simulink model "FFT_Analysis_Synthesis_VHDL"  (R2020a)
settings: Solver=FixedStepDiscrete  StartTime=0.0  StopTime=1  RelTol=1e-3
InitFcn:
  | sm_callback_init
StopFcn:
  | sm_callback_stop
values from neighbouring files (symbols this model uses):
  mp = sm_init_control_signals(mp)    [sm_callback_init.m]    (also in sm_callback_stop.m = sm_stop_verify(mp))
libraries: hdlsllib x32, simulink x12, dsphdlxfrm x4, dspsigops x2
(part 2 of 2)

== system FFT_Analysis_Synthesis_VHDL/dataplane/FFT_Analysis_Synthesis_Left/Analysis/FFT Frame Buffering/FFT_pulse_gen/Wait_for_data_to_start ==
  note: Frame pulses don't start
      | coming through until
      | circular buffer has data.
  note: Counter starts a zero and counts number of frame pulses.
      | Counter remains enabled while frame count is less than 4.
      | As soon as the counter reaches 4, it is disabled, which then
      | enables the frame pulses to pass through.
  note: Frame_Pulse
      | will pass through
      | when enabled
  note: Number of Frames
      | to wait before starting
  note: Start performing FFTs after enough data has filled the circular buffer.
      | This is due to the fact that we don't want the read pointer (addr_B)
      | to catch up with the write pointer (addr_A) because if it does,
      | the DPRAM will throw an assertion error.
  note: Enable signal that that indicates
      | that FFTs can start since there is
      | data in the buffer.
  Frame_Pulse : Inport
  Bitwise Operator : simulink/Logic and Bit Operations/Bitwise Operator  logicop=NOT  UseBitMask=off  BitMask=bin2dec('11011001')  BitMaskRealWorld=Stored Integer
  Compare To Constant : simulink/Logic and Bit Operations/Compare To Constant  relop=<  const=4  OutDataTypeStr=boolean
  Initial_frame_count : hdlsllib/Sources/HDL Counter  CountType=Count limited  CountInit=0  CountStep=1  CountMax=4  CountFromType=Specify  CountFrom=0  CountResetPort=off  CountLoadPort=off  CountEnbPort=on  CountDirPort=off  CountDataType=Unsigned  CountWordLen=5  CountFracLen=0  CountSampTime=1
  Logical Operator : Logic  AllPortsSameDT=off  OutDataTypeStr=boolean
  Logical Operator1 : Logic  AllPortsSameDT=off  OutDataTypeStr=boolean
  FFT_Frame_Start : Outport  VectorParamsAs1DForOutWhenUnconnected=off
  Enable_FFT_Frames : Outport  Port=2  VectorParamsAs1DForOutWhenUnconnected=off
  wires:
  Logical Operator1/1 -> FFT_Frame_Start/1
  Frame_Pulse/1 -> Logical Operator/2, Logical Operator1/1
  Initial_frame_count/1 -> Compare To Constant/1
  Logical Operator/1 -> Initial_frame_count/1
  Compare To Constant/1 -> Bitwise Operator/1, Logical Operator/1
  Bitwise Operator/1 -> Enable_FFT_Frames/1, Logical Operator1/2

== system FFT_Analysis_Synthesis_VHDL/dataplane/FFT_Analysis_Synthesis_Left/Analysis/FFT Frame Buffering/addr_B_gen/addr_B_gen_enable ==
  note: Signal that is enabled while
      | counting [0 FFT_size-1]
  note: Frame_index is the count [0 FFT_size-1]
      | that is used to lookup the window value
      | being applied to the streaming sample.
  note: This counter specifies where the FFT starts
      | in the circular buffer.  It increments by FFT/4
      | samples when it receives a start pulse.
  note: The start pulse resets the counter that counts
      | from zero to FFT_size-1.  Upon reaching FFT_size
      | the counter is disabled.  While the counter is enabled,
      | the enable signal tells the FFT engine that the data streaming
      | to it is valid.
  start : Inport
  B_Enable_Counter : hdlsllib/Sources/HDL Counter  CountType=Count limited  CountInit=0  CountStep=1  CountMax=mp.FFT_size  CountFromType=Specify  CountFrom=0  CountResetPort=on  CountLoadPort=off  CountEnbPort=on  CountDirPort=off  CountDataType=Unsigned  CountWordLen=mp.DPRAM1_address_size  CountFracLen=0  CountSampTime=1
  Constant5 : Constant  Value=mp.FFT_size  OutDataTypeStr=fixdt(0,mp.FFT_size_Nbits,0)  SampleTime=mp.Ts/mp.SysRate_Upsample_Factor
  Relational Operator : RelationalOperator  Operator=<=  OutDataTypeStr=boolean  ZeroCross=off  RndMeth=Nearest
  Start_Address_Counter : hdlsllib/Sources/HDL Counter  CountType=Free running  CountInit=0  CountStep=mp.FFT_frame_shift  CountMax=25  CountFromType=Initial value  CountFrom=0  CountResetPort=off  CountLoadPort=off  CountEnbPort=on  CountDirPort=off  CountDataType=Unsigned  CountWordLen=mp.DPRAM1_address_size  CountFracLen=0  CountSampTime=1
  enable_B : Outport  VectorParamsAs1DForOutWhenUnconnected=off
  Start_Address : Outport  Port=2  VectorParamsAs1DForOutWhenUnconnected=off
  Frame_Index : Outport  Port=3  VectorParamsAs1DForOutWhenUnconnected=off
  wires:
  Relational Operator/1 -> enable_B/1, B_Enable_Counter/2
  Constant5/1 -> Relational Operator/2
  B_Enable_Counter/1 -> Frame_Index/1, Relational Operator/1
  start/1 -> B_Enable_Counter/1, Start_Address_Counter/1
  Start_Address_Counter/1 -> Start_Address/1

== system FFT_Analysis_Synthesis_VHDL/dataplane/FFT_Analysis_Synthesis_Left/Frequency_Domain_Processing/Apply_Complex_Gains/FFT_Filter_Coefficients/FFT_ROM_Indexing ==
  note: When the index is FFT_size/2, we want the
      | index to be zero.
  note: Count from 0 to FFT_size
  note: Reverse direction of
      | count when count
      | is FFT_size/2
  note: Count from 0 to FFT_size/2 and then back down to 0.
      | We are assuming the gains are conjugate symmetric
      | so we only need to store the first half in the ROM
      | and look up again for negative frequencies.
  valid : Inport
  Bitwise Operator : simulink/Logic and Bit Operations/Bitwise Operator  logicop=NOT  UseBitMask=off  BitMask=bin2dec('11011001')  BitMaskRealWorld=Stored Integer
  Constant : Constant  Value=0  OutDataTypeStr=fixdt(0,mp.FFT_size_Nbits,0)  SampleTime=mp.Ts/mp.SysRate_Upsample_Factor
  Constant5 : Constant  Value=mp.FFT_size_half  OutDataTypeStr=fixdt(0,mp.FFT_size_Nbits,0)  SampleTime=mp.Ts/mp.SysRate_Upsample_Factor
  FFT_count : hdlsllib/Sources/HDL Counter  CountType=Free running  CountInit=0  CountStep=1  CountMax=25  CountFromType=Initial value  CountFrom=0  CountResetPort=on  CountLoadPort=off  CountEnbPort=on  CountDirPort=off  CountDataType=Unsigned  CountWordLen=mp.FFT_size_Nbits  CountFracLen=0  CountSampTime=1
  Relational Operator : RelationalOperator  Operator=<  OutDataTypeStr=boolean  ZeroCross=off  RndMeth=Nearest
  Relational Operator1 : RelationalOperator  Operator=~=  OutDataTypeStr=boolean  ZeroCross=off  RndMeth=Nearest
  Switch : Switch  Criteria=u2 > Threshold
  counter_gain_index : hdlsllib/Sources/HDL Counter  CountType=Free running  CountInit=0  CountStep=1  CountMax=25  CountFromType=Initial value  CountFrom=0  CountResetPort=on  CountLoadPort=off  CountEnbPort=on  CountDirPort=on  CountDataType=Unsigned  CountWordLen=mp.FFT_size_Nbits  CountFracLen=0  CountSampTime=1
  ROM_index : Outport
  wires:
  Relational Operator/1 -> counter_gain_index/3
  Bitwise Operator/1 -> FFT_count/1, counter_gain_index/1
  Relational Operator1/1 -> Switch/2
  FFT_count/1 -> Relational Operator/1
  valid/1 -> FFT_count/2, counter_gain_index/2, Bitwise Operator/1
  Constant5/1 -> Relational Operator1/2, Relational Operator/2
  counter_gain_index/1 -> Switch/1, Relational Operator1/1
  Constant/1 -> Switch/3
  Switch/1 -> ROM_index/1

== system FFT_Analysis_Synthesis_VHDL/dataplane/FFT_Analysis_Synthesis_Left/Frequency_Domain_Processing/Apply_Complex_Gains/FFT_Filter_Coefficients/Filter_ROM_Choice ==
  select : Inport
  Index : Inport  Port=2
  Complex_Gains_1_ROM : Subsystem
  Complex_Gains_2_ROM : Subsystem
  Complex_Gains_3_ROM : Subsystem
  Complex_Gains_4_ROM : Subsystem
  Multiport Switch : MultiPortSwitch  DataPortOrder=Zero-based contiguous  Inputs=4  zeroidx=on
  filter_gains : Outport
  wires:
  Multiport Switch/1 -> filter_gains/1
  Index/1 -> Complex_Gains_1_ROM/1(Index), Complex_Gains_2_ROM/1(Index), Complex_Gains_3_ROM/1(Index), Complex_Gains_4_ROM/1(Index)
  Complex_Gains_4_ROM/1(gains) -> Multiport Switch/5
  Complex_Gains_1_ROM/1(gains) -> Multiport Switch/2
  Complex_Gains_2_ROM/1(gains) -> Multiport Switch/3
  select/1 -> Multiport Switch/1
  Complex_Gains_3_ROM/1(gains) -> Multiport Switch/4

== system FFT_Analysis_Synthesis_VHDL/dataplane/FFT_Analysis_Synthesis_Right/Analysis/FFT Frame Buffering/FFT_pulse_gen/FFT_Frame_Pulse_Gen ==
  note: Create a FFT frame pulse that happens every FFT_size/4 samples.
      | We do this by watching when an appropriate subset of the counter bits
      | become zero.
  "counter_value " : Inport
  Bit Slice : hdlsllib/Logic and Bit Operations/Bit Slice  lidx=log2(mp.FFT_frame_shift)-1  ridx=0
      settings: SourceProductBaseCode=SL
  Compare To Zero : simulink/Logic and Bit Operations/Compare To Zero  relop===  OutDataTypeStr=boolean
  Frame_Pulse : Outport  VectorParamsAs1DForOutWhenUnconnected=off
  wires:
  "counter_value "/1 -> Bit Slice/1
  Compare To Zero/1 -> Frame_Pulse/1
  Bit Slice/1 -> Compare To Zero/1

== system FFT_Analysis_Synthesis_VHDL/dataplane/FFT_Analysis_Synthesis_Right/Analysis/FFT Frame Buffering/FFT_pulse_gen/Wait_for_data_to_start ==
  note: Frame pulses don't start
      | coming through until
      | circular buffer has data.
  note: Counter starts a zero and counts number of frame pulses.
      | Counter remains enabled while frame count is less than 4.
      | As soon as the counter reaches 4, it is disabled, which then
      | enables the frame pulses to pass through.
  note: Frame_Pulse
      | will pass through
      | when enabled
  note: Number of Frames
      | to wait before starting
  note: Start performing FFTs after enough data has filled the circular buffer.
      | This is due to the fact that we don't want the read pointer (addr_B)
      | to catch up with the write pointer (addr_A) because if it does,
      | the DPRAM will throw an assertion error.
  note: Enable signal that that indicates
      | that FFTs can start since there is
      | data in the buffer.
  Frame_Pulse : Inport
  Bitwise Operator : simulink/Logic and Bit Operations/Bitwise Operator  logicop=NOT  UseBitMask=off  BitMask=bin2dec('11011001')  BitMaskRealWorld=Stored Integer
  Compare To Constant : simulink/Logic and Bit Operations/Compare To Constant  relop=<  const=4  OutDataTypeStr=boolean
  Initial_frame_count : hdlsllib/Sources/HDL Counter  CountType=Count limited  CountInit=0  CountStep=1  CountMax=4  CountFromType=Specify  CountFrom=0  CountResetPort=off  CountLoadPort=off  CountEnbPort=on  CountDirPort=off  CountDataType=Unsigned  CountWordLen=5  CountFracLen=0  CountSampTime=1
  Logical Operator : Logic  AllPortsSameDT=off  OutDataTypeStr=boolean
  Logical Operator1 : Logic  AllPortsSameDT=off  OutDataTypeStr=boolean
  FFT_Frame_Start : Outport  VectorParamsAs1DForOutWhenUnconnected=off
  Enable_FFT_Frames : Outport  Port=2  VectorParamsAs1DForOutWhenUnconnected=off
  wires:
  Logical Operator1/1 -> FFT_Frame_Start/1
  Frame_Pulse/1 -> Logical Operator/2, Logical Operator1/1
  Initial_frame_count/1 -> Compare To Constant/1
  Logical Operator/1 -> Initial_frame_count/1
  Compare To Constant/1 -> Bitwise Operator/1, Logical Operator/1
  Bitwise Operator/1 -> Enable_FFT_Frames/1, Logical Operator1/2

== system FFT_Analysis_Synthesis_VHDL/dataplane/FFT_Analysis_Synthesis_Right/Analysis/FFT Frame Buffering/addr_B_gen/addr_B_gen_enable ==
  note: Signal that is enabled while
      | counting [0 FFT_size-1]
  note: Frame_index is the count [0 FFT_size-1]
      | that is used to lookup the window value
      | being applied to the streaming sample.
  note: This counter specifies where the FFT starts
      | in the circular buffer.  It increments by FFT/4
      | samples when it receives a start pulse.
  note: The start pulse resets the counter that counts
      | from zero to FFT_size-1.  Upon reaching FFT_size
      | the counter is disabled.  While the counter is enabled,
      | the enable signal tells the FFT engine that the data streaming
      | to it is valid.
  start : Inport
  B_Enable_Counter : hdlsllib/Sources/HDL Counter  CountType=Count limited  CountInit=0  CountStep=1  CountMax=mp.FFT_size  CountFromType=Specify  CountFrom=0  CountResetPort=on  CountLoadPort=off  CountEnbPort=on  CountDirPort=off  CountDataType=Unsigned  CountWordLen=mp.DPRAM1_address_size  CountFracLen=0  CountSampTime=1
  Constant5 : Constant  Value=mp.FFT_size  OutDataTypeStr=fixdt(0,mp.FFT_size_Nbits,0)  SampleTime=mp.Ts/mp.SysRate_Upsample_Factor
  Relational Operator : RelationalOperator  Operator=<=  OutDataTypeStr=boolean  ZeroCross=off  RndMeth=Nearest
  Start_Address_Counter : hdlsllib/Sources/HDL Counter  CountType=Free running  CountInit=0  CountStep=mp.FFT_frame_shift  CountMax=25  CountFromType=Initial value  CountFrom=0  CountResetPort=off  CountLoadPort=off  CountEnbPort=on  CountDirPort=off  CountDataType=Unsigned  CountWordLen=mp.DPRAM1_address_size  CountFracLen=0  CountSampTime=1
  enable_B : Outport  VectorParamsAs1DForOutWhenUnconnected=off
  Start_Address : Outport  Port=2  VectorParamsAs1DForOutWhenUnconnected=off
  Frame_Index : Outport  Port=3  VectorParamsAs1DForOutWhenUnconnected=off
  wires:
  Relational Operator/1 -> enable_B/1, B_Enable_Counter/2
  Constant5/1 -> Relational Operator/2
  B_Enable_Counter/1 -> Frame_Index/1, Relational Operator/1
  start/1 -> B_Enable_Counter/1, Start_Address_Counter/1
  Start_Address_Counter/1 -> Start_Address/1

== system FFT_Analysis_Synthesis_VHDL/dataplane/FFT_Analysis_Synthesis_Right/Frequency_Domain_Processing/Apply_Complex_Gains/FFT_Filter_Coefficients/FFT_ROM_Indexing ==
  note: When the index is FFT_size/2, we want the
      | index to be zero.
  note: Count from 0 to FFT_size
  note: Reverse direction of
      | count when count
      | is FFT_size/2
  note: Count from 0 to FFT_size/2 and then back down to 0.
      | We are assuming the gains are conjugate symmetric
      | so we only need to store the first half in the ROM
      | and look up again for negative frequencies.
  valid : Inport
  Bitwise Operator : simulink/Logic and Bit Operations/Bitwise Operator  logicop=NOT  UseBitMask=off  BitMask=bin2dec('11011001')  BitMaskRealWorld=Stored Integer
  Constant : Constant  Value=0  OutDataTypeStr=fixdt(0,mp.FFT_size_Nbits,0)  SampleTime=mp.Ts/mp.SysRate_Upsample_Factor
  Constant5 : Constant  Value=mp.FFT_size_half  OutDataTypeStr=fixdt(0,mp.FFT_size_Nbits,0)  SampleTime=mp.Ts/mp.SysRate_Upsample_Factor
  FFT_count : hdlsllib/Sources/HDL Counter  CountType=Free running  CountInit=0  CountStep=1  CountMax=25  CountFromType=Initial value  CountFrom=0  CountResetPort=on  CountLoadPort=off  CountEnbPort=on  CountDirPort=off  CountDataType=Unsigned  CountWordLen=mp.FFT_size_Nbits  CountFracLen=0  CountSampTime=1
  Relational Operator : RelationalOperator  Operator=<  OutDataTypeStr=boolean  ZeroCross=off  RndMeth=Nearest
  Relational Operator1 : RelationalOperator  Operator=~=  OutDataTypeStr=boolean  ZeroCross=off  RndMeth=Nearest
  Switch : Switch  Criteria=u2 > Threshold
  counter_gain_index : hdlsllib/Sources/HDL Counter  CountType=Free running  CountInit=0  CountStep=1  CountMax=25  CountFromType=Initial value  CountFrom=0  CountResetPort=on  CountLoadPort=off  CountEnbPort=on  CountDirPort=on  CountDataType=Unsigned  CountWordLen=mp.FFT_size_Nbits  CountFracLen=0  CountSampTime=1
  ROM_index : Outport
  wires:
  Relational Operator/1 -> counter_gain_index/3
  Bitwise Operator/1 -> FFT_count/1, counter_gain_index/1
  Relational Operator1/1 -> Switch/2
  FFT_count/1 -> Relational Operator/1
  valid/1 -> FFT_count/2, counter_gain_index/2, Bitwise Operator/1
  Constant5/1 -> Relational Operator1/2, Relational Operator/2
  counter_gain_index/1 -> Switch/1, Relational Operator1/1
  Constant/1 -> Switch/3
  Switch/1 -> ROM_index/1

== system FFT_Analysis_Synthesis_VHDL/dataplane/FFT_Analysis_Synthesis_Right/Frequency_Domain_Processing/Apply_Complex_Gains/FFT_Filter_Coefficients/Filter_ROM_Choice ==
  select : Inport
  Index : Inport  Port=2
  Complex_Gains_1_ROM : Subsystem
  Complex_Gains_2_ROM : Subsystem
  Complex_Gains_3_ROM : Subsystem
  Complex_Gains_4_ROM : Subsystem
  Multiport Switch : MultiPortSwitch  DataPortOrder=Zero-based contiguous  Inputs=4  zeroidx=on
  filter_gains : Outport
  wires:
  Multiport Switch/1 -> filter_gains/1
  Index/1 -> Complex_Gains_1_ROM/1(Index), Complex_Gains_2_ROM/1(Index), Complex_Gains_3_ROM/1(Index), Complex_Gains_4_ROM/1(Index)
  Complex_Gains_4_ROM/1(gains) -> Multiport Switch/5
  Complex_Gains_1_ROM/1(gains) -> Multiport Switch/2
  Complex_Gains_2_ROM/1(gains) -> Multiport Switch/3
  select/1 -> Multiport Switch/1
  Complex_Gains_3_ROM/1(gains) -> Multiport Switch/4

== system FFT_Analysis_Synthesis_VHDL/dataplane/FFT_Analysis_Synthesis_Left/Frequency_Domain_Processing/Apply_Complex_Gains/FFT_Filter_Coefficients/Filter_ROM_Choice/Complex_Gains_1_ROM ==
  Index : Inport
  Gains_ROM_imag : Subsystem
  Gains_ROM_real : Subsystem
  Real-Imag to Complex : RealImagToComplex
  gains : Outport
  wires:
  Gains_ROM_imag/1(gain_value_imag) -> Real-Imag to Complex/2
  Index/1 -> Gains_ROM_imag/1(Index), Gains_ROM_real/1(Index)
  Gains_ROM_real/1(gain_value_real) -> Real-Imag to Complex/1
  Real-Imag to Complex/1 -> gains/1

== system FFT_Analysis_Synthesis_VHDL/dataplane/FFT_Analysis_Synthesis_Left/Frequency_Domain_Processing/Apply_Complex_Gains/FFT_Filter_Coefficients/Filter_ROM_Choice/Complex_Gains_2_ROM ==
  Index : Inport
  Gains_ROM_imag : Subsystem
  Gains_ROM_real : Subsystem
  Real-Imag to Complex : RealImagToComplex
  gains : Outport
  wires:
  Gains_ROM_imag/1(gain_value_imag) -> Real-Imag to Complex/2
  Index/1 -> Gains_ROM_imag/1(Index), Gains_ROM_real/1(Index)
  Gains_ROM_real/1(gain_value_real) -> Real-Imag to Complex/1
  Real-Imag to Complex/1 -> gains/1

== system FFT_Analysis_Synthesis_VHDL/dataplane/FFT_Analysis_Synthesis_Left/Frequency_Domain_Processing/Apply_Complex_Gains/FFT_Filter_Coefficients/Filter_ROM_Choice/Complex_Gains_3_ROM ==
  Index : Inport
  Gains_ROM_imag : Subsystem
  Gains_ROM_real : Subsystem
  Real-Imag to Complex : RealImagToComplex
  gains : Outport
  wires:
  Gains_ROM_imag/1(gain_value_imag) -> Real-Imag to Complex/2
  Index/1 -> Gains_ROM_imag/1(Index), Gains_ROM_real/1(Index)
  Gains_ROM_real/1(gain_value_real) -> Real-Imag to Complex/1
  Real-Imag to Complex/1 -> gains/1

== system FFT_Analysis_Synthesis_VHDL/dataplane/FFT_Analysis_Synthesis_Left/Frequency_Domain_Processing/Apply_Complex_Gains/FFT_Filter_Coefficients/Filter_ROM_Choice/Complex_Gains_4_ROM ==
  Index : Inport
  Gains_ROM_imag : Subsystem
  Gains_ROM_real : Subsystem
  Real-Imag to Complex : RealImagToComplex
  gains : Outport
  wires:
  Gains_ROM_imag/1(gain_value_imag) -> Real-Imag to Complex/2
  Index/1 -> Gains_ROM_imag/1(Index), Gains_ROM_real/1(Index)
  Gains_ROM_real/1(gain_value_real) -> Real-Imag to Complex/1
  Real-Imag to Complex/1 -> gains/1

== system FFT_Analysis_Synthesis_VHDL/dataplane/FFT_Analysis_Synthesis_Right/Frequency_Domain_Processing/Apply_Complex_Gains/FFT_Filter_Coefficients/Filter_ROM_Choice/Complex_Gains_1_ROM ==
  Index : Inport
  Gains_ROM_imag : Subsystem
  Gains_ROM_real : Subsystem
  Real-Imag to Complex : RealImagToComplex
  gains : Outport
  wires:
  Gains_ROM_imag/1(gain_value_imag) -> Real-Imag to Complex/2
  Index/1 -> Gains_ROM_imag/1(Index), Gains_ROM_real/1(Index)
  Gains_ROM_real/1(gain_value_real) -> Real-Imag to Complex/1
  Real-Imag to Complex/1 -> gains/1

== system FFT_Analysis_Synthesis_VHDL/dataplane/FFT_Analysis_Synthesis_Right/Frequency_Domain_Processing/Apply_Complex_Gains/FFT_Filter_Coefficients/Filter_ROM_Choice/Complex_Gains_2_ROM ==
  Index : Inport
  Gains_ROM_imag : Subsystem
  Gains_ROM_real : Subsystem
  Real-Imag to Complex : RealImagToComplex
  gains : Outport
  wires:
  Gains_ROM_imag/1(gain_value_imag) -> Real-Imag to Complex/2
  Index/1 -> Gains_ROM_imag/1(Index), Gains_ROM_real/1(Index)
  Gains_ROM_real/1(gain_value_real) -> Real-Imag to Complex/1
  Real-Imag to Complex/1 -> gains/1

== system FFT_Analysis_Synthesis_VHDL/dataplane/FFT_Analysis_Synthesis_Right/Frequency_Domain_Processing/Apply_Complex_Gains/FFT_Filter_Coefficients/Filter_ROM_Choice/Complex_Gains_3_ROM ==
  Index : Inport
  Gains_ROM_imag : Subsystem
  Gains_ROM_real : Subsystem
  Real-Imag to Complex : RealImagToComplex
  gains : Outport
  wires:
  Gains_ROM_imag/1(gain_value_imag) -> Real-Imag to Complex/2
  Index/1 -> Gains_ROM_imag/1(Index), Gains_ROM_real/1(Index)
  Gains_ROM_real/1(gain_value_real) -> Real-Imag to Complex/1
  Real-Imag to Complex/1 -> gains/1

== system FFT_Analysis_Synthesis_VHDL/dataplane/FFT_Analysis_Synthesis_Right/Frequency_Domain_Processing/Apply_Complex_Gains/FFT_Filter_Coefficients/Filter_ROM_Choice/Complex_Gains_4_ROM ==
  Index : Inport
  Gains_ROM_imag : Subsystem
  Gains_ROM_real : Subsystem
  Real-Imag to Complex : RealImagToComplex
  gains : Outport
  wires:
  Gains_ROM_imag/1(gain_value_imag) -> Real-Imag to Complex/2
  Index/1 -> Gains_ROM_imag/1(Index), Gains_ROM_real/1(Index)
  Gains_ROM_real/1(gain_value_real) -> Real-Imag to Complex/1
  Real-Imag to Complex/1 -> gains/1

== system FFT_Analysis_Synthesis_VHDL/dataplane/FFT_Analysis_Synthesis_Left/Frequency_Domain_Processing/Apply_Complex_Gains/FFT_Filter_Coefficients/Filter_ROM_Choice/Complex_Gains_1_ROM/Gains_ROM_imag ==
  Index : Inport
  Lookup Table : Lookup_n-D  NumberOfTableDimensions=1  BreakpointsForDimension1=[0:mp.FFT_size_half-1]  IndexSearchMethod=Evenly spaced points  Table=mp.fft_gains_1_imag  InterpMethod=Flat  ExtrapMethod=Clip  DiagnosticForOutOfRangeInput=Error  UseLastTableValue=on  OutDataTypeStr=fixdt(1,mp.W_bits,mp.F_bits)  RndMeth=Simplest  InputSameDT=on
  Unit Delay : UnitDelay  SampleTime=-1  HasFrameUpgradeWarning=on
  gain_value_imag : Outport  VectorParamsAs1DForOutWhenUnconnected=off
  wires:
  Unit Delay/1 -> gain_value_imag/1
  Index/1 -> Lookup Table/1
  Lookup Table/1 -> Unit Delay/1

== system FFT_Analysis_Synthesis_VHDL/dataplane/FFT_Analysis_Synthesis_Left/Frequency_Domain_Processing/Apply_Complex_Gains/FFT_Filter_Coefficients/Filter_ROM_Choice/Complex_Gains_1_ROM/Gains_ROM_real ==
  Index : Inport
  Lookup Table : Lookup_n-D  NumberOfTableDimensions=1  BreakpointsForDimension1=[0:mp.FFT_size_half-1]  IndexSearchMethod=Evenly spaced points  Table=mp.fft_gains_1_real  InterpMethod=Flat  ExtrapMethod=Clip  DiagnosticForOutOfRangeInput=Error  UseLastTableValue=on  OutDataTypeStr=fixdt(1,mp.W_bits,mp.F_bits)  RndMeth=Simplest  InputSameDT=on
  Unit Delay : UnitDelay  SampleTime=-1  HasFrameUpgradeWarning=on
  gain_value_real : Outport  VectorParamsAs1DForOutWhenUnconnected=off
  wires:
  Unit Delay/1 -> gain_value_real/1
  Index/1 -> Lookup Table/1
  Lookup Table/1 -> Unit Delay/1

== system FFT_Analysis_Synthesis_VHDL/dataplane/FFT_Analysis_Synthesis_Left/Frequency_Domain_Processing/Apply_Complex_Gains/FFT_Filter_Coefficients/Filter_ROM_Choice/Complex_Gains_2_ROM/Gains_ROM_imag ==
  Index : Inport
  Lookup Table : Lookup_n-D  NumberOfTableDimensions=1  BreakpointsForDimension1=[0:mp.FFT_size_half-1]  IndexSearchMethod=Evenly spaced points  Table=mp.fft_gains_2_imag  InterpMethod=Flat  ExtrapMethod=Clip  DiagnosticForOutOfRangeInput=Error  UseLastTableValue=on  OutDataTypeStr=fixdt(1,mp.W_bits,mp.F_bits)  RndMeth=Simplest  InputSameDT=on
  Unit Delay : UnitDelay  SampleTime=-1  HasFrameUpgradeWarning=on
  gain_value_imag : Outport  VectorParamsAs1DForOutWhenUnconnected=off
  wires:
  Unit Delay/1 -> gain_value_imag/1
  Index/1 -> Lookup Table/1
  Lookup Table/1 -> Unit Delay/1

== system FFT_Analysis_Synthesis_VHDL/dataplane/FFT_Analysis_Synthesis_Left/Frequency_Domain_Processing/Apply_Complex_Gains/FFT_Filter_Coefficients/Filter_ROM_Choice/Complex_Gains_2_ROM/Gains_ROM_real ==
  Index : Inport
  Lookup Table : Lookup_n-D  NumberOfTableDimensions=1  BreakpointsForDimension1=[0:mp.FFT_size_half-1]  IndexSearchMethod=Evenly spaced points  Table=mp.fft_gains_2_real  InterpMethod=Flat  ExtrapMethod=Clip  DiagnosticForOutOfRangeInput=Error  UseLastTableValue=on  OutDataTypeStr=fixdt(1,mp.W_bits,mp.F_bits)  RndMeth=Simplest  InputSameDT=on
  Unit Delay : UnitDelay  SampleTime=-1  HasFrameUpgradeWarning=on
  gain_value_real : Outport  VectorParamsAs1DForOutWhenUnconnected=off
  wires:
  Unit Delay/1 -> gain_value_real/1
  Index/1 -> Lookup Table/1
  Lookup Table/1 -> Unit Delay/1

== system FFT_Analysis_Synthesis_VHDL/dataplane/FFT_Analysis_Synthesis_Left/Frequency_Domain_Processing/Apply_Complex_Gains/FFT_Filter_Coefficients/Filter_ROM_Choice/Complex_Gains_3_ROM/Gains_ROM_imag ==
  Index : Inport
  Lookup Table : Lookup_n-D  NumberOfTableDimensions=1  BreakpointsForDimension1=[0:mp.FFT_size_half-1]  IndexSearchMethod=Evenly spaced points  Table=mp.fft_gains_3_imag  InterpMethod=Flat  ExtrapMethod=Clip  DiagnosticForOutOfRangeInput=Error  UseLastTableValue=on  OutDataTypeStr=fixdt(1,mp.W_bits,mp.F_bits)  RndMeth=Simplest  InputSameDT=on
  Unit Delay : UnitDelay  SampleTime=-1  HasFrameUpgradeWarning=on
  gain_value_imag : Outport  VectorParamsAs1DForOutWhenUnconnected=off
  wires:
  Unit Delay/1 -> gain_value_imag/1
  Index/1 -> Lookup Table/1
  Lookup Table/1 -> Unit Delay/1

== system FFT_Analysis_Synthesis_VHDL/dataplane/FFT_Analysis_Synthesis_Left/Frequency_Domain_Processing/Apply_Complex_Gains/FFT_Filter_Coefficients/Filter_ROM_Choice/Complex_Gains_3_ROM/Gains_ROM_real ==
  Index : Inport
  Lookup Table : Lookup_n-D  NumberOfTableDimensions=1  BreakpointsForDimension1=[0:mp.FFT_size_half-1]  IndexSearchMethod=Evenly spaced points  Table=mp.fft_gains_3_real  InterpMethod=Flat  ExtrapMethod=Clip  DiagnosticForOutOfRangeInput=Error  UseLastTableValue=on  OutDataTypeStr=fixdt(1,mp.W_bits,mp.F_bits)  RndMeth=Simplest  InputSameDT=on
  Unit Delay : UnitDelay  SampleTime=-1  HasFrameUpgradeWarning=on
  gain_value_real : Outport  VectorParamsAs1DForOutWhenUnconnected=off
  wires:
  Unit Delay/1 -> gain_value_real/1
  Index/1 -> Lookup Table/1
  Lookup Table/1 -> Unit Delay/1

== system FFT_Analysis_Synthesis_VHDL/dataplane/FFT_Analysis_Synthesis_Left/Frequency_Domain_Processing/Apply_Complex_Gains/FFT_Filter_Coefficients/Filter_ROM_Choice/Complex_Gains_4_ROM/Gains_ROM_imag ==
  Index : Inport
  Lookup Table : Lookup_n-D  NumberOfTableDimensions=1  BreakpointsForDimension1=[0:mp.FFT_size_half-1]  IndexSearchMethod=Evenly spaced points  Table=mp.fft_gains_4_imag  InterpMethod=Flat  ExtrapMethod=Clip  DiagnosticForOutOfRangeInput=Error  UseLastTableValue=on  OutDataTypeStr=fixdt(1,mp.W_bits,mp.F_bits)  RndMeth=Simplest  InputSameDT=on
  Unit Delay : UnitDelay  SampleTime=-1  HasFrameUpgradeWarning=on
  gain_value_imag : Outport  VectorParamsAs1DForOutWhenUnconnected=off
  wires:
  Unit Delay/1 -> gain_value_imag/1
  Index/1 -> Lookup Table/1
  Lookup Table/1 -> Unit Delay/1

== system FFT_Analysis_Synthesis_VHDL/dataplane/FFT_Analysis_Synthesis_Left/Frequency_Domain_Processing/Apply_Complex_Gains/FFT_Filter_Coefficients/Filter_ROM_Choice/Complex_Gains_4_ROM/Gains_ROM_real ==
  Index : Inport
  Lookup Table : Lookup_n-D  NumberOfTableDimensions=1  BreakpointsForDimension1=[0:mp.FFT_size_half-1]  IndexSearchMethod=Evenly spaced points  Table=mp.fft_gains_4_real  InterpMethod=Flat  ExtrapMethod=Clip  DiagnosticForOutOfRangeInput=Error  UseLastTableValue=on  OutDataTypeStr=fixdt(1,mp.W_bits,mp.F_bits)  RndMeth=Simplest  InputSameDT=on
  Unit Delay : UnitDelay  SampleTime=-1  HasFrameUpgradeWarning=on
  gain_value_real : Outport  VectorParamsAs1DForOutWhenUnconnected=off
  wires:
  Unit Delay/1 -> gain_value_real/1
  Index/1 -> Lookup Table/1
  Lookup Table/1 -> Unit Delay/1

== system FFT_Analysis_Synthesis_VHDL/dataplane/FFT_Analysis_Synthesis_Right/Frequency_Domain_Processing/Apply_Complex_Gains/FFT_Filter_Coefficients/Filter_ROM_Choice/Complex_Gains_1_ROM/Gains_ROM_imag ==
  Index : Inport
  Lookup Table : Lookup_n-D  NumberOfTableDimensions=1  BreakpointsForDimension1=[0:mp.FFT_size_half-1]  IndexSearchMethod=Evenly spaced points  Table=mp.fft_gains_1_imag  InterpMethod=Flat  ExtrapMethod=Clip  DiagnosticForOutOfRangeInput=Error  UseLastTableValue=on  OutDataTypeStr=fixdt(1,mp.W_bits,mp.F_bits)  RndMeth=Simplest  InputSameDT=on
  Unit Delay : UnitDelay  SampleTime=-1  HasFrameUpgradeWarning=on
  gain_value_imag : Outport  VectorParamsAs1DForOutWhenUnconnected=off
  wires:
  Unit Delay/1 -> gain_value_imag/1
  Index/1 -> Lookup Table/1
  Lookup Table/1 -> Unit Delay/1

== system FFT_Analysis_Synthesis_VHDL/dataplane/FFT_Analysis_Synthesis_Right/Frequency_Domain_Processing/Apply_Complex_Gains/FFT_Filter_Coefficients/Filter_ROM_Choice/Complex_Gains_1_ROM/Gains_ROM_real ==
  Index : Inport
  Lookup Table : Lookup_n-D  NumberOfTableDimensions=1  BreakpointsForDimension1=[0:mp.FFT_size_half-1]  IndexSearchMethod=Evenly spaced points  Table=mp.fft_gains_1_real  InterpMethod=Flat  ExtrapMethod=Clip  DiagnosticForOutOfRangeInput=Error  UseLastTableValue=on  OutDataTypeStr=fixdt(1,mp.W_bits,mp.F_bits)  RndMeth=Simplest  InputSameDT=on
  Unit Delay : UnitDelay  SampleTime=-1  HasFrameUpgradeWarning=on
  gain_value_real : Outport  VectorParamsAs1DForOutWhenUnconnected=off
  wires:
  Unit Delay/1 -> gain_value_real/1
  Index/1 -> Lookup Table/1
  Lookup Table/1 -> Unit Delay/1

== system FFT_Analysis_Synthesis_VHDL/dataplane/FFT_Analysis_Synthesis_Right/Frequency_Domain_Processing/Apply_Complex_Gains/FFT_Filter_Coefficients/Filter_ROM_Choice/Complex_Gains_2_ROM/Gains_ROM_imag ==
  Index : Inport
  Lookup Table : Lookup_n-D  NumberOfTableDimensions=1  BreakpointsForDimension1=[0:mp.FFT_size_half-1]  IndexSearchMethod=Evenly spaced points  Table=mp.fft_gains_2_imag  InterpMethod=Flat  ExtrapMethod=Clip  DiagnosticForOutOfRangeInput=Error  UseLastTableValue=on  OutDataTypeStr=fixdt(1,mp.W_bits,mp.F_bits)  RndMeth=Simplest  InputSameDT=on
  Unit Delay : UnitDelay  SampleTime=-1  HasFrameUpgradeWarning=on
  gain_value_imag : Outport  VectorParamsAs1DForOutWhenUnconnected=off
  wires:
  Unit Delay/1 -> gain_value_imag/1
  Index/1 -> Lookup Table/1
  Lookup Table/1 -> Unit Delay/1

== system FFT_Analysis_Synthesis_VHDL/dataplane/FFT_Analysis_Synthesis_Right/Frequency_Domain_Processing/Apply_Complex_Gains/FFT_Filter_Coefficients/Filter_ROM_Choice/Complex_Gains_2_ROM/Gains_ROM_real ==
  Index : Inport
  Lookup Table : Lookup_n-D  NumberOfTableDimensions=1  BreakpointsForDimension1=[0:mp.FFT_size_half-1]  IndexSearchMethod=Evenly spaced points  Table=mp.fft_gains_2_real  InterpMethod=Flat  ExtrapMethod=Clip  DiagnosticForOutOfRangeInput=Error  UseLastTableValue=on  OutDataTypeStr=fixdt(1,mp.W_bits,mp.F_bits)  RndMeth=Simplest  InputSameDT=on
  Unit Delay : UnitDelay  SampleTime=-1  HasFrameUpgradeWarning=on
  gain_value_real : Outport  VectorParamsAs1DForOutWhenUnconnected=off
  wires:
  Unit Delay/1 -> gain_value_real/1
  Index/1 -> Lookup Table/1
  Lookup Table/1 -> Unit Delay/1

== system FFT_Analysis_Synthesis_VHDL/dataplane/FFT_Analysis_Synthesis_Right/Frequency_Domain_Processing/Apply_Complex_Gains/FFT_Filter_Coefficients/Filter_ROM_Choice/Complex_Gains_3_ROM/Gains_ROM_imag ==
  Index : Inport
  Lookup Table : Lookup_n-D  NumberOfTableDimensions=1  BreakpointsForDimension1=[0:mp.FFT_size_half-1]  IndexSearchMethod=Evenly spaced points  Table=mp.fft_gains_3_imag  InterpMethod=Flat  ExtrapMethod=Clip  DiagnosticForOutOfRangeInput=Error  UseLastTableValue=on  OutDataTypeStr=fixdt(1,mp.W_bits,mp.F_bits)  RndMeth=Simplest  InputSameDT=on
  Unit Delay : UnitDelay  SampleTime=-1  HasFrameUpgradeWarning=on
  gain_value_imag : Outport  VectorParamsAs1DForOutWhenUnconnected=off
  wires:
  Unit Delay/1 -> gain_value_imag/1
  Index/1 -> Lookup Table/1
  Lookup Table/1 -> Unit Delay/1

== system FFT_Analysis_Synthesis_VHDL/dataplane/FFT_Analysis_Synthesis_Right/Frequency_Domain_Processing/Apply_Complex_Gains/FFT_Filter_Coefficients/Filter_ROM_Choice/Complex_Gains_3_ROM/Gains_ROM_real ==
  Index : Inport
  Lookup Table : Lookup_n-D  NumberOfTableDimensions=1  BreakpointsForDimension1=[0:mp.FFT_size_half-1]  IndexSearchMethod=Evenly spaced points  Table=mp.fft_gains_3_real  InterpMethod=Flat  ExtrapMethod=Clip  DiagnosticForOutOfRangeInput=Error  UseLastTableValue=on  OutDataTypeStr=fixdt(1,mp.W_bits,mp.F_bits)  RndMeth=Simplest  InputSameDT=on
  Unit Delay : UnitDelay  SampleTime=-1  HasFrameUpgradeWarning=on
  gain_value_real : Outport  VectorParamsAs1DForOutWhenUnconnected=off
  wires:
  Unit Delay/1 -> gain_value_real/1
  Index/1 -> Lookup Table/1
  Lookup Table/1 -> Unit Delay/1

== system FFT_Analysis_Synthesis_VHDL/dataplane/FFT_Analysis_Synthesis_Right/Frequency_Domain_Processing/Apply_Complex_Gains/FFT_Filter_Coefficients/Filter_ROM_Choice/Complex_Gains_4_ROM/Gains_ROM_imag ==
  Index : Inport
  Lookup Table : Lookup_n-D  NumberOfTableDimensions=1  BreakpointsForDimension1=[0:mp.FFT_size_half-1]  IndexSearchMethod=Evenly spaced points  Table=mp.fft_gains_4_imag  InterpMethod=Flat  ExtrapMethod=Clip  DiagnosticForOutOfRangeInput=Error  UseLastTableValue=on  OutDataTypeStr=fixdt(1,mp.W_bits,mp.F_bits)  RndMeth=Simplest  InputSameDT=on
  Unit Delay : UnitDelay  SampleTime=-1  HasFrameUpgradeWarning=on
  gain_value_imag : Outport  VectorParamsAs1DForOutWhenUnconnected=off
  wires:
  Unit Delay/1 -> gain_value_imag/1
  Index/1 -> Lookup Table/1
  Lookup Table/1 -> Unit Delay/1

== system FFT_Analysis_Synthesis_VHDL/dataplane/FFT_Analysis_Synthesis_Right/Frequency_Domain_Processing/Apply_Complex_Gains/FFT_Filter_Coefficients/Filter_ROM_Choice/Complex_Gains_4_ROM/Gains_ROM_real ==
  Index : Inport
  Lookup Table : Lookup_n-D  NumberOfTableDimensions=1  BreakpointsForDimension1=[0:mp.FFT_size_half-1]  IndexSearchMethod=Evenly spaced points  Table=mp.fft_gains_4_real  InterpMethod=Flat  ExtrapMethod=Clip  DiagnosticForOutOfRangeInput=Error  UseLastTableValue=on  OutDataTypeStr=fixdt(1,mp.W_bits,mp.F_bits)  RndMeth=Simplest  InputSameDT=on
  Unit Delay : UnitDelay  SampleTime=-1  HasFrameUpgradeWarning=on
  gain_value_real : Outport  VectorParamsAs1DForOutWhenUnconnected=off
  wires:
  Unit Delay/1 -> gain_value_real/1
  Index/1 -> Lookup Table/1
  Lookup Table/1 -> Unit Delay/1

== matlab function FFT_Analysis_Synthesis_VHDL/dataplane/FFT_Analysis_Synthesis_Left/Synthesis/Overlap_and_Add/FIFO_Write_Select ==
  data: fifo_counter input; valid_1 output; valid_signal input; valid_2 output; valid_3 output; valid_4 output
function [valid_1, valid_2, valid_3, valid_4] = fcn(fifo_counter, valid_signal)
%#codegen



switch fifo_counter
    case 0
        valid_1 = valid_signal;
        valid_2 = false;
        valid_3 = false;
        valid_4 = false;
    case 1
        valid_1 = false;
        valid_2 = valid_signal;
        valid_3 = false;
        valid_4 = false;
    case 2
        valid_1 = false;
        valid_2 = false;
        valid_3 = valid_signal;
        valid_4 = false;
    case 3
        valid_1 = false;
        valid_2 = false;
        valid_3 = false;
        valid_4 = valid_signal;
    otherwise
        valid_1 = false;
        valid_2 = false;
        valid_3 = false;
        valid_4 = false;
       
end

== matlab function FFT_Analysis_Synthesis_VHDL/dataplane/FFT_Analysis_Synthesis_Left/Synthesis/Overlap_and_Add/fifo_state_machine ==
  data: valid input; pop output
function pop = fifo_state_machine(valid)
%#codegen

state_valid_low = 0;
state_valid_high = 1;
state_assert_pop = 2;

persistent current_state;
if isempty(current_state)
    current_state = state_valid_low;
end

switch(current_state)
    case state_valid_low

        pop = false;
        
        if valid
            current_state = state_valid_high;
        else
            current_state = state_valid_low;
        end
        
    case state_valid_high
        
        pop = false;
        
        if valid
            current_state = state_valid_high;
        else
            current_state = state_assert_pop;
        end
        
    case state_assert_pop
        
        pop = true;
        
        current_state = state_assert_pop;
        
    otherwise
        
        pop = false;
        
end

== stateflow chart FFT_Analysis_Synthesis_VHDL/dataplane/FFT_Analysis_Synthesis_Right/Synthesis/Overlap_and_Add/Chart ==
  settings: stateMachineType=MOORE_MACHINE  executeAtInitialization=1
  state valid_high
    Pop_Valid=fi(0,0,1,0);
  state Pop_assert
    Pop_Valid=fi(1,0,1,0);
  state valid_low
    Pop_Valid=fi(0,0,1,0);
  state Start_up
    Pop_Valid=fi(0,0,1,0);
  (default) -> Start_up
  Start_up -> valid_low : [valid == 0]
  valid_high -> Pop_assert [order 1] : [valid == 0]
  valid_low -> valid_high [order 1] : [valid == 1]
  valid_low -> valid_low [order 2] : [valid == 0]
  valid_high -> valid_high [order 2] : [valid == 1]
  data: valid input; Pop_Valid output

== stateflow chart FFT_Analysis_Synthesis_VHDL/dataplane/FFT_Analysis_Synthesis_Right/Synthesis/Overlap_and_Add/Chart1 ==
  settings: stateMachineType=MOORE_MACHINE  executeAtInitialization=1
  state valid_high
    Pop_Valid=fi(0,0,1,0);
  state Pop_assert
    Pop_Valid=fi(1,0,1,0);
  state valid_low
    Pop_Valid=fi(0,0,1,0);
  state Start_up
    Pop_Valid=fi(0,0,1,0);
  (default) -> Start_up
  Start_up -> valid_low : [valid == 0]
  valid_high -> Pop_assert [order 1] : [valid == 0]
  valid_low -> valid_high [order 1] : [valid == 1]
  valid_low -> valid_low [order 2] : [valid == 0]
  valid_high -> valid_high [order 2] : [valid == 1]
  data: valid input; Pop_Valid output

== stateflow chart FFT_Analysis_Synthesis_VHDL/dataplane/FFT_Analysis_Synthesis_Right/Synthesis/Overlap_and_Add/Chart2 ==
  settings: stateMachineType=MOORE_MACHINE  executeAtInitialization=1
  state valid_high
    Pop_Valid=fi(0,0,1,0);
  state Pop_assert
    Pop_Valid=fi(1,0,1,0);
  state valid_low
    Pop_Valid=fi(0,0,1,0);
  state Start_up
    Pop_Valid=fi(0,0,1,0);
  (default) -> Start_up
  Start_up -> valid_low : [valid == 0]
  valid_high -> Pop_assert [order 1] : [valid == 0]
  valid_low -> valid_high [order 1] : [valid == 1]
  valid_low -> valid_low [order 2] : [valid == 0]
  valid_high -> valid_high [order 2] : [valid == 1]
  data: valid input; Pop_Valid output

== stateflow chart FFT_Analysis_Synthesis_VHDL/dataplane/FFT_Analysis_Synthesis_Right/Synthesis/Overlap_and_Add/Chart3 ==
  settings: stateMachineType=MOORE_MACHINE  executeAtInitialization=1
  state valid_high
    Pop_Valid=fi(0,0,1,0);
  state Pop_assert
    Pop_Valid=fi(1,0,1,0);
  state valid_low
    Pop_Valid=fi(0,0,1,0);
  state Start_up
    Pop_Valid=fi(0,0,1,0);
  (default) -> Start_up
  Start_up -> valid_low : [valid == 0]
  valid_high -> Pop_assert [order 1] : [valid == 0]
  valid_low -> valid_high [order 1] : [valid == 1]
  valid_low -> valid_low [order 2] : [valid == 0]
  valid_high -> valid_high [order 2] : [valid == 1]
  data: valid input; Pop_Valid output

== matlab function FFT_Analysis_Synthesis_VHDL/dataplane/FFT_Analysis_Synthesis_Left/Synthesis/Overlap_and_Add/fifo_state_machine1 ==
  data: valid input; pop output
function pop = fifo_state_machine(valid)
%#codegen

state_valid_low = 0;
state_valid_high = 1;
state_assert_pop = 2;

persistent current_state;
if isempty(current_state)
    current_state = state_valid_low;
end

switch(current_state)
    case state_valid_low

        pop = false;
        
        if valid
            current_state = state_valid_high;
        else
            current_state = state_valid_low;
        end
        
    case state_valid_high
        
        pop = false;
        
        if valid
            current_state = state_valid_high;
        else
            current_state = state_assert_pop;
        end
        
    case state_assert_pop
        
        pop = true;
        
        current_state = state_assert_pop;
        
    otherwise
        
        pop = false;
        
end

== matlab function FFT_Analysis_Synthesis_VHDL/dataplane/FFT_Analysis_Synthesis_Left/Synthesis/Overlap_and_Add/fifo_state_machine2 ==
  data: valid input; pop output
function pop = fifo_state_machine(valid)
%#codegen

state_valid_low = 0;
state_valid_high = 1;
state_assert_pop = 2;

persistent current_state;
if isempty(current_state)
    current_state = state_valid_low;
end

switch(current_state)
    case state_valid_low

        pop = false;
        
        if valid
            current_state = state_valid_high;
        else
            current_state = state_valid_low;
        end
        
    case state_valid_high
        
        pop = false;
        
        if valid
            current_state = state_valid_high;
        else
            current_state = state_assert_pop;
        end
        
    case state_assert_pop
        
        pop = true;
        
        current_state = state_assert_pop;
        
    otherwise
        
        pop = false;
        
end

== matlab function FFT_Analysis_Synthesis_VHDL/dataplane/FFT_Analysis_Synthesis_Left/Synthesis/Overlap_and_Add/fifo_state_machine3 ==
  data: valid input; pop output
function pop = fifo_state_machine(valid)
%#codegen

state_valid_low = 0;
state_valid_high = 1;
state_assert_pop = 2;

persistent current_state;
if isempty(current_state)
    current_state = state_valid_low;
end

switch(current_state)
    case state_valid_low

        pop = false;
        
        if valid
            current_state = state_valid_high;
        else
            current_state = state_valid_low;
        end
        
    case state_valid_high
        
        pop = false;
        
        if valid
            current_state = state_valid_high;
        else
            current_state = state_assert_pop;
        end
        
    case state_assert_pop
        
        pop = true;
        
        current_state = state_assert_pop;
        
    otherwise
        
        pop = false;
        
end

== matlab function FFT_Analysis_Synthesis_VHDL/dataplane/FFT_Analysis_Synthesis_Right/Synthesis/Overlap_and_Add/FIFO_Write_Select ==
  data: fifo_counter input; valid_1 output; valid_signal input; valid_2 output; valid_3 output; valid_4 output
function [valid_1, valid_2, valid_3, valid_4] = fcn(fifo_counter, valid_signal)
%#codegen



switch fifo_counter
    case 0
        valid_1 = valid_signal;
        valid_2 = false;
        valid_3 = false;
        valid_4 = false;
    case 1
        valid_1 = false;
        valid_2 = valid_signal;
        valid_3 = false;
        valid_4 = false;
    case 2
        valid_1 = false;
        valid_2 = false;
        valid_3 = valid_signal;
        valid_4 = false;
    case 3
        valid_1 = false;
        valid_2 = false;
        valid_3 = false;
        valid_4 = valid_signal;
    otherwise
        valid_1 = false;
        valid_2 = false;
        valid_3 = false;
        valid_4 = false;
       
end
